simulink model "ad9361_sim"  (R2015b)
settings: Solver=ode45  StartTime=0.0  StopTime=Inf  RelTol=1e-3
libraries: simulink x2, dspsrcs4 x1
settings Model: Creator=ACozma  LastModifiedBy=ACozma
settings DataIOCC: SaveFormat=Array
settings DebuggingCC: UnderspecifiedInitializationDetection=Classic  MergeDetectMultiDrivingBlocksExec=none  SolverPrmCheckMsg=warning
settings HardwareCC: ProdBitPerPointer=32  ProdLargestAtomicFloat=None  ProdIntDivRoundTo=Undefined  ProdEndianess=Unspecified  ProdWordSize=32  ProdHWDeviceType=32-bit Generic
settings GRTTargetCC: GeneratePreprocessorConditionals=Disable all
settings ConfigComp: CovModelRefEnable=Off  CovSFcnEnable=off

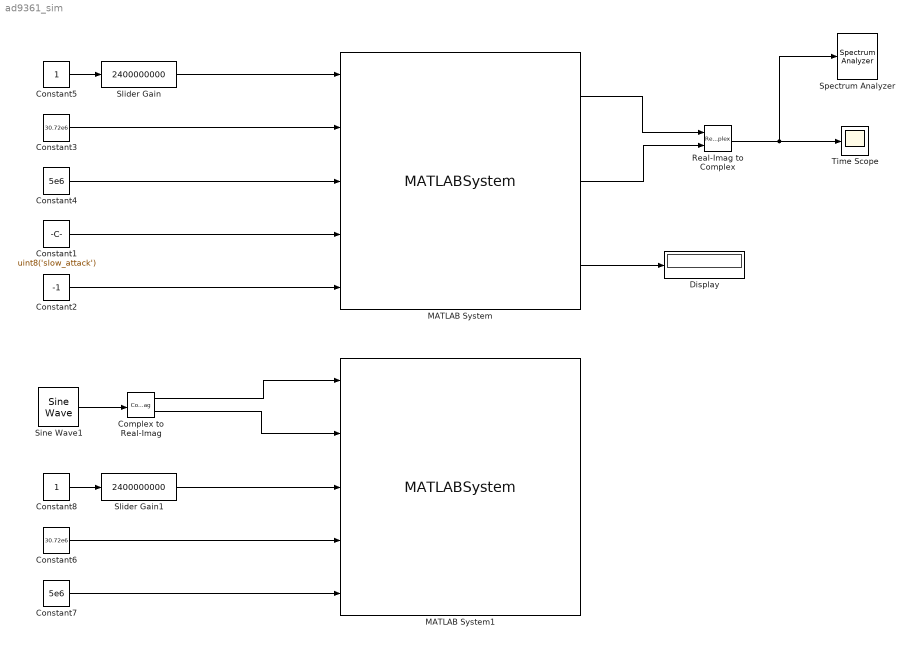
== system ad9361_sim ==
  Complex to Real-Imag : ComplexToRealImag
  Constant1 : Constant  Value=uint8('slow_attack')  SampleTime=-1
  Constant2 : Constant  Value=-1  SampleTime=-1
  Constant3 : Constant  Value=30.72e6  SampleTime=-1
  Constant4 : Constant  Value=5e6  SampleTime=-1
  Constant5 : Constant  SampleTime=-1
  Constant6 : Constant  Value=30.72e6  SampleTime=-1
  Constant7 : Constant  Value=5e6  SampleTime=-1
  Constant8 : Constant  SampleTime=-1
  Display : Display
  MATLAB System : MATLABSystem  DialogController=sysobjdialog.BlockDynDialog  System=iio_sys_obj  ip_address=10.50.1.122  dev_name=ad9361_rx  in_ch_no=0  in_ch_size=32768  out_ch_no=2  out_ch_size=32768  SimulateUsing=Interpreted execution
      mask Type: iio_sys_obj
      mask Display:
      | disp('ad9361_rx');
      | port_label('input',1,'RX_LO_FREQ');
      | port_label('input',2,'RX_SAMPLING_FREQ');
      | port_label('input',3,'RX_RF_BANDWIDTH');
      | port_label('input',4,'RX1_GAIN_MODE');
      | port_label('input',5,'RX1_GAIN');
      | port_label('output',1,'DATA_OUT1');
      | port_label('output',2,'DATA_OUT2');
      | port_label('output',3,'RX1_RSSI');
  MATLAB System1 : MATLABSystem  DialogController=sysobjdialog.BlockDynDialog  System=iio_sys_obj  ip_address=10.50.1.122  dev_name=ad9361_tx  in_ch_no=2  in_ch_size=32768  out_ch_no=0  out_ch_size=32768  SimulateUsing=Interpreted execution
      mask Type: iio_sys_obj
      mask Display:
      | disp('ad9361_tx');
      | port_label('input',1,'DATA_IN1');
      | port_label('input',2,'DATA_IN2');
      | port_label('input',3,'TX_LO_FREQ');
      | port_label('input',4,'TX_SAMPLING_FREQ');
      | port_label('input',5,'TX_RF_BANDWIDTH');
  Real-Imag to Complex : RealImagToComplex
  Sine Wave1 : dspsrcs4/Sine Wave  Amplitude=3200  Frequency=1.4e6  Phase=0  SampleMode=Discrete  OutComplex=Complex  CompMethod=Trigonometric fcn  TableSize=Speed  SampleTime=1/30.72e6  SamplesPerFrame=32768  ResetState=Catch up to simulation time  OutputFrames=on  dataType=double  wordLen=16  udDataType=sfix(16)  fracBitsMode=Best precision  numFracBits=15  OutDataTypeStr=double  LastOutDataTypeStr=double
  Slider Gain : simulink/Math Operations/Slider Gain  low=200000  gain=2400000000  high=6000000000
  Slider Gain1 : simulink/Math Operations/Slider Gain  low=200000  gain=2400000000  high=6000000000
  Spectrum Analyzer : SpectrumAnalyzer
  Time Scope : Scope
  wires:
  Constant5/1 -> Slider Gain/1
  Constant8/1 -> Slider Gain1/1
  MATLAB System/1 -> Real-Imag to Complex/1
  MATLAB System/2 -> Real-Imag to Complex/2
  Real-Imag to Complex/1 -> Spectrum Analyzer/1, Time Scope/1
  MATLAB System/3 -> Display/1
  Slider Gain/1 -> MATLAB System/1
  Constant3/1 -> MATLAB System/2
  Constant4/1 -> MATLAB System/3
  Constant1/1 -> MATLAB System/4
  Constant2/1 -> MATLAB System/5
  Slider Gain1/1 -> MATLAB System1/3
  Constant6/1 -> MATLAB System1/4
  Constant7/1 -> MATLAB System1/5
  Complex to Real-Imag/1 -> MATLAB System1/1
  Complex to Real-Imag/2 -> MATLAB System1/2
  Sine Wave1/1 -> Complex to Real-Imag/1
